simulink model "absorber_model_2"  (R2022a)
settings: Solver=VariableStepAuto  StartTime=0.0  StopTime=60  RelTol=1e-3
settings Model: Creator=Home  LastModifiedBy=Home

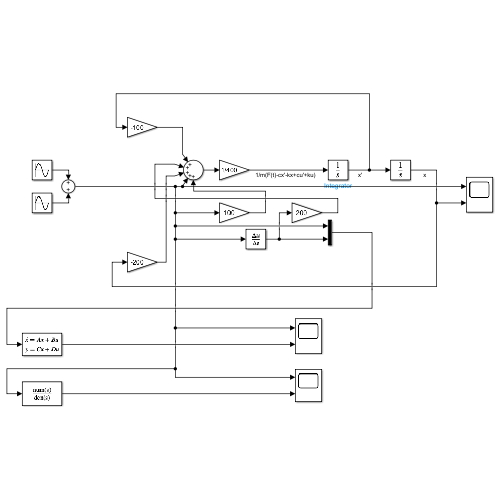
[thumbnail: Simulink's stored preview of the top-level diagram]
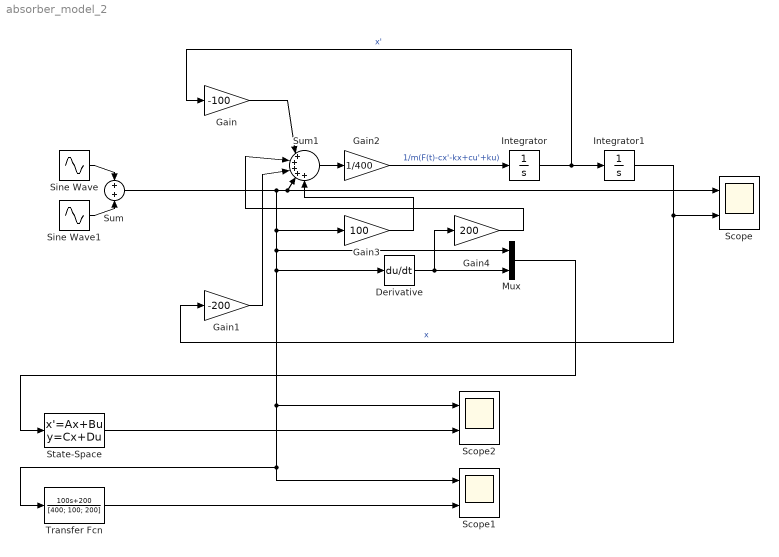
== system absorber_model_2 ==
  Derivative : Derivative
  Gain : Gain  Gain=-100
  Gain1 : Gain  Gain=-200
  Gain2 : Gain  Gain=1/400
  Gain3 : Gain  Gain=100
  Gain4 : Gain  Gain=200
  Integrator : Integrator
  Integrator1 : Integrator
  Mux : Mux  Inputs=2
  Scope : Scope  NumInputPorts=2
  Scope1 : Scope  NumInputPorts=2
  Scope2 : Scope  NumInputPorts=2
  Sine Wave : Sin  Frequency=0.195  SampleTime=0
  Sine Wave1 : Sin  Frequency=20  SampleTime=0
  State-Space : StateSpace  A=[0 1; -200/400 -100/400]  B=[0 0; 200/400 100/400]  C=[1 0]  D=[0 0]  InitialCondition=0  ParameterTunability=Unconstrained
  Sum : Sum
  Sum1 : Sum  Inputs=|+++++
  Transfer Fcn : TransferFcn  Numerator=[100, 200]  Denominator=[400; 100; 200]
  wires:
  Sine Wave/1 -> Sum/1
  Sine Wave1/1 -> Sum/2
  Gain/1 -> Sum1/1
  Gain1/1 -> Sum1/3
  Sum1/1 -> Gain2/1
  Integrator1/1 -> Gain1/1, Scope/2  "x"
  Integrator/1 -> Gain/1, Integrator1/1  "x'"
  State-Space/1 -> Scope2/2
  Transfer Fcn/1 -> Scope1/2
  Gain2/1 -> Integrator/1  "1/m(F(t)-cx'-kx+cu'+ku)"
  Mux/1 -> State-Space/1
  Gain3/1 -> Sum1/5
  Derivative/1 -> Gain4/1, Mux/2
  Gain4/1 -> Sum1/2
  Sum/1 -> Scope/1, Sum1/4, Scope1/1, Transfer Fcn/1, Scope2/1, Derivative/1, Mux/1, Gain3/1
